simulink model "control_loop_v01"  (R2022b)
settings: Solver=FixedStepAuto  StartTime=0.0  StopTime=10.0  FixedStep=0.05  RelTol=1e-3
libraries: simulink x1
settings Model: Creator=lricc  LastModifiedBy=lricc

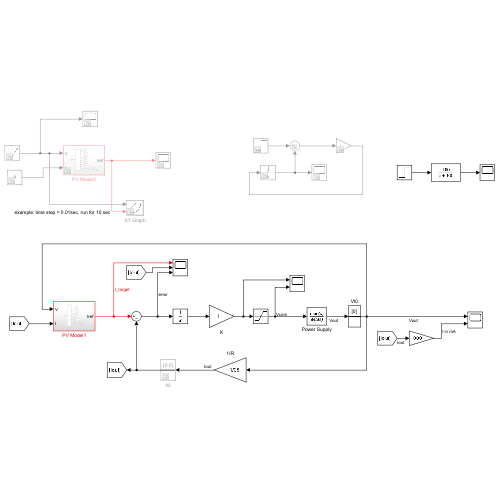
[thumbnail: Simulink's stored preview of the top-level diagram]
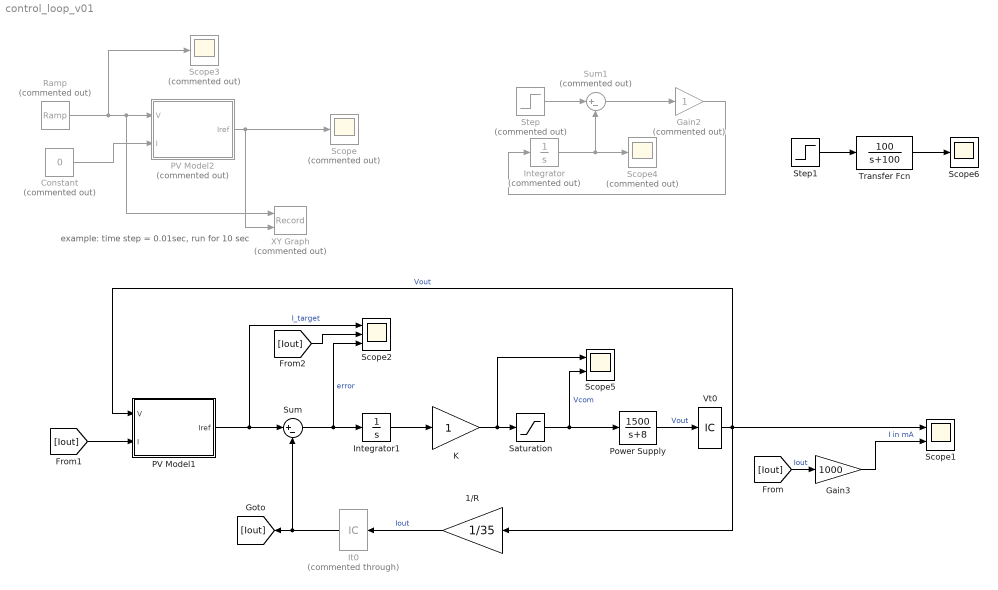
== system control_loop_v01 ==
  note: example: time step = 0.01sec, run for 10 sec
  1/R : Gain  Gain=1/35
  Constant : Constant  Commented=on  Value=0
  Gain2 : Gain  Commented=on
  Gain3 : Gain  Gain=1000
  Integrator : Integrator  Commented=on
  Integrator1 : Integrator
  It0 : InitialCondition  Commented=through  Value=0.0
  K : Gain
  PV Model1 : Subsystem
  PV Model2 : Subsystem  Commented=on
  Power Supply : TransferFcn  Numerator=[1500]  Denominator=[1 8]
  Ramp : simulink/Sources/Ramp  Commented=on  slope=1.8  start=0  InitialOutput=0
  Saturation : Saturate  UpperLimit=18.8  LowerLimit=0
  Scope : Scope  Commented=on
  Scope1 : Scope  NumInputPorts=2
  Scope2 : Scope  NumInputPorts=3
  Scope3 : Scope  Commented=on
  Scope4 : Scope  Commented=on
  Scope5 : Scope  NumInputPorts=2
  Scope6 : Scope
  Step : Step  Commented=on  SampleTime=0
  Step1 : Step  SampleTime=0
  Sum : Sum  Inputs=|+-
  Sum1 : Sum  Commented=on  Inputs=|+-
  Transfer Fcn : TransferFcn  Numerator=[100]  Denominator=[1 100]
  Vt0 : InitialCondition  Value=0
  XY Graph : Record  Commented=on  FileSettingsInternal="{\"entries\":[{\"content\":{\"excelSettings\":{\"content\":{},\"type\":\"Streamout.ExcelSettings\"}},\"type\":\"Streamout.FileSettingStorage\",\"uuid\":\"914085eb-a8da-4e62-ba7d-c15c726b2b54\"}],\"packageUris\":[\"http://schema.mathworks.com/mf0/streamout_blocks/R2020a\"],\"version\":\"1.0\"}"  Layout=[1 1]  SignalsInternal="{\"entries\":[{\"content\":{\"signals\":[{\"content\":{\"blockPath\":[\"control_loop_v01/XY Graph\"],\"channel\":[],\"dimensions\":[1],\"domain\":\"control_loop_v01/XY Graph\",\"lineColor\":\"#a2142f\",\"plots\":[1],\"port\":1,\"sid\":[],\"signalID\":8,\"signalName\":\"Ramp\"},\"type\":\"RecordBlkView.Signal\",\"uuid\":\"80a78c32-fe05-49ae-b46e-e4b479ed4a3a\"},{\"content\":{\"blockPath\":[\"control_loop_v01/XY Graph\"],\"channel\":[],\"dimensions\":[1],\"domain\":\"control_loop_v01/XY Graph\",\"lineColor\":\"#139fff\",\"plots\":[1],\"port\":2,\"sid\":[],\"signalID\":11,\"signalName\":\"PV Model2\"},\"type\":\"RecordBlkView.Signal\",\"uuid\":\"f08b557e-ddef-419a-8417-18afe662ca76\"}]},\"type\":\"RecordBlkView.InputSignals\",\"uuid\":\"ba897e66-074b-46d2-a743-d3e4d107ee1a\"}],\"packageUris\":[\"http://schema.mathworks.com/mf0/streamout_blocks/R2020a\"],\"version\":\"1.0\"}"  VisualizationBindings="{\"xyplotplugin\":{\"info\":[{\"series\":[{\"bindingParametersList\":[{\"parameter\":\"X-Axis\",\"signalID\":8,\"signalName\":\"Ramp\"},{\"parameter\":\"Y-Axis\",\"signalID\":11,\"signalName\":\"PV Model2\"}],\"seriesID\":26463}],\"subplotID\":1}]}}"  CompatibilityTag=XY
  wires:
  Sum/1 -> Scope2/3, Integrator1/1  "error"
  PV Model1/1(Iref) -> Scope2/1, Sum/1  "I_target"
  1/R/1 -> It0/1  "Iout"
  K/1 -> Scope5/1, Saturation/1
  PV Model2/1(Iref) -> XY Graph/2, Scope/1
  Ramp/1 -> XY Graph/1, PV Model2/1(V), Scope3/1
  Constant/1 -> PV Model2/2(I)
  [Iout] -> PV Model1/2(I)
  [Iout] -> Gain3/1  "Iout"
  Step/1 -> Sum1/1
  Integrator/1 -> Scope4/1, Sum1/2
  Sum1/1 -> Gain2/1
  Gain2/1 -> Integrator/1
  Integrator1/1 -> K/1
  Saturation/1 -> Scope5/2, Power Supply/1  "Vcom"
  Gain3/1 -> Scope1/2  "I in mA"
  Step1/1 -> Transfer Fcn/1
  Transfer Fcn/1 -> Scope6/1
  Power Supply/1 -> Vt0/1  "Vout"
  Vt0/1 -> PV Model1/1(V), 1/R/1, Scope1/1  "Vout"
  It0/1 -> Sum/2, [Iout]
  [Iout] -> Scope2/2

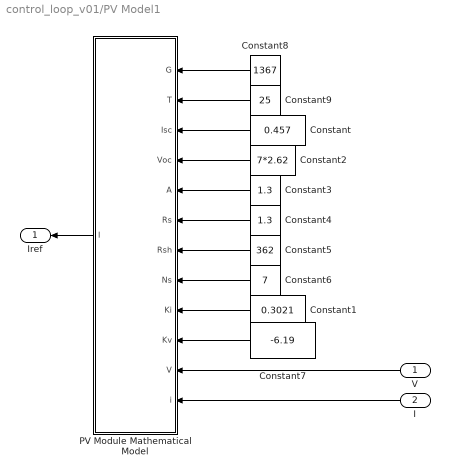
== system control_loop_v01/PV Model1 ==
  V : Inport
  I : Inport  Port=2
  Constant : Constant  Value=0.457
  Constant1 : Constant  Value=0.3021
  Constant2 : Constant  Value=7*2.62
  Constant3 : Constant  Value=1.3
  Constant4 : Constant  Value=1.3
  Constant5 : Constant  Value=362
  Constant6 : Constant  Value=7
  Constant7 : Constant  Value=-6.19
  Constant8 : Constant  Value=1367
  Constant9 : Constant  Value=25
  PV Module Mathematical Model : MATLAB Function  TreatAsAtomicUnit=on
  Iref : Outport
  wires:
  Constant/1 -> PV Module Mathematical Model/3(Isc)
  Constant7/1 -> PV Module Mathematical Model/10(Kv)
  Constant5/1 -> PV Module Mathematical Model/7(Rsh)
  Constant6/1 -> PV Module Mathematical Model/8(Ns)
  Constant1/1 -> PV Module Mathematical Model/9(Ki)
  Constant8/1 -> PV Module Mathematical Model/1(G)
  Constant4/1 -> PV Module Mathematical Model/6(Rs)
  Constant2/1 -> PV Module Mathematical Model/4(Voc)
  Constant9/1 -> PV Module Mathematical Model/2(T)
  Constant3/1 -> PV Module Mathematical Model/5(A)
  PV Module Mathematical Model/1(I) -> Iref/1
  I/1 -> PV Module Mathematical Model/12(i)
  V/1 -> PV Module Mathematical Model/11(V)

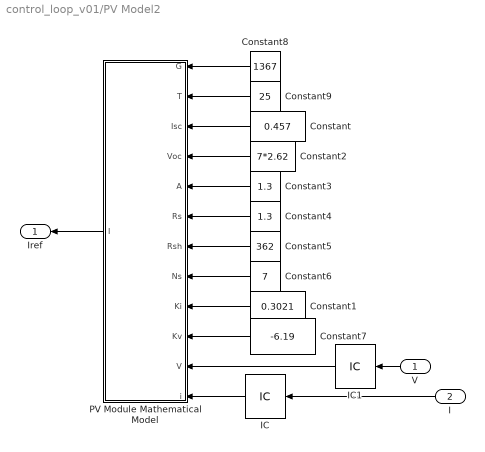
== system control_loop_v01/PV Model2 ==
  V : Inport
  I : Inport  Port=2
  Constant : Constant  Value=0.457
  Constant1 : Constant  Value=0.3021
  Constant2 : Constant  Value=7*2.62
  Constant3 : Constant  Value=1.3
  Constant4 : Constant  Value=1.3
  Constant5 : Constant  Value=362
  Constant6 : Constant  Value=7
  Constant7 : Constant  Value=-6.19
  Constant8 : Constant  Value=1367
  Constant9 : Constant  Value=25
  IC : InitialCondition  Value=0.4
  IC1 : InitialCondition  Value=15
  PV Module Mathematical Model : MATLAB Function  TreatAsAtomicUnit=on
  Iref : Outport
  wires:
  Constant/1 -> PV Module Mathematical Model/3(Isc)
  Constant7/1 -> PV Module Mathematical Model/10(Kv)
  Constant5/1 -> PV Module Mathematical Model/7(Rsh)
  Constant6/1 -> PV Module Mathematical Model/8(Ns)
  Constant1/1 -> PV Module Mathematical Model/9(Ki)
  Constant8/1 -> PV Module Mathematical Model/1(G)
  Constant4/1 -> PV Module Mathematical Model/6(Rs)
  Constant2/1 -> PV Module Mathematical Model/4(Voc)
  Constant9/1 -> PV Module Mathematical Model/2(T)
  Constant3/1 -> PV Module Mathematical Model/5(A)
  PV Module Mathematical Model/1(I) -> Iref/1
  I/1 -> IC/1
  IC/1 -> PV Module Mathematical Model/12(i)
  V/1 -> IC1/1
  IC1/1 -> PV Module Mathematical Model/11(V)

== matlab function control_loop_v01/PV Model1/PV Module Mathematical Model ==
  data: G input; T input; Isc input; Voc input; A input; Rs input; Rsh input; Ns input; Ki input; Kv input; V input; i input; I output
function I = fcn(G,T,Isc,Voc,A,Rs,Rsh,Ns,Ki,Kv,V,i)
    
    q = 1.6e-19;                          % Electron charge
    k = 1.38e-23;                         % Boltzmann constant
    Tcell = 273+T;                        % Cell temperature in Kelvin
    vt=(A*k*Tcell*Ns)/q;                  % Thermal voltage Equation(5)
        
    Isc_T = Isc+((Isc*(Ki/1000))*(T-25));  % Isc temperature coef Equation(6)
    Voc_T = Voc+((Voc*(Kv/1000))*(T-25));  % Voc temperature coef Equation(7)
    Is = Isc_T/(exp(Voc_T/vt)-1);         % Reverse saturation current Equation(8)
    Iph = Isc_T*(G/1367);                 % Photon current Equation(9)
    
    % Single diode model output current Equation(4)
    %I = Iph-(Is*(exp((V+(i*Rs))/vt)-1))-((V+(i*Rs))/Rsh);
    I = Iph - (Is * (exp((V + (i * Rs)) / vt) - 1))    - ((V/Ns   + (i * Rs)) / Rsh);
    if  I< 0.0 
    I = 0;
    end
end

== matlab function control_loop_v01/PV Model2/PV Module Mathematical Model ==
  data: G input; T input; Isc input; Voc input; A input; Rs input; Rsh input; Ns input; Ki input; Kv input; V input; i input; I output
function I = fcn(G,T,Isc,Voc,A,Rs,Rsh,Ns,Ki,Kv,V,i)
    
    q = 1.6e-19;                          % Electron charge
    k = 1.38e-23;                         % Boltzmann constant
    Tcell = 273+T;                        % Cell temperature in Kelvin
    vt=(A*k*Tcell*Ns)/q;                  % Thermal voltage Equation(5)
        
    Isc_T = Isc+((Isc*(Ki/1000))*(T-25));  % Isc temperature coef Equation(6)
    Voc_T = Voc+((Voc*(Kv/1000))*(T-25));  % Voc temperature coef Equation(7)
    Is = Isc_T/(exp(Voc_T/vt)-1);         % Reverse saturation current Equation(8)
    Iph = Isc_T*(G/1367);                 % Photon current Equation(9)
    
    % Single diode model output current Equation(4)
    %I = Iph-(Is*(exp((V+(i*Rs))/vt)-1))-((V+(i*Rs))/Rsh);
    I = Iph - (Is * (exp((V + (i * Rs)) / vt) - 1))    - ((V/Ns   + (i * Rs)) / Rsh);
    if  I< 0.0 
    I = 0;
    end
end
